simulink model "MotorModelSteadyStateCharacteristics"  (R2015b)
settings: Solver=VariableStepAuto  StartTime=0.0  StopTime=2000  RelTol=1e-4
values from neighbouring files (symbols this model uses):
  R_winding = Vdc_nom/I_stall    (= 0.16724738676)    [MotorModel_Mabuchi_RS_540.m]
  Vdc = 9.6    [MotorModel_Mabuchi_RS_540.m]    (also in Params.m)
libraries: simulink x7, LocalLib x1
settings Model: Creator=jje  LastModifiedBy=jje

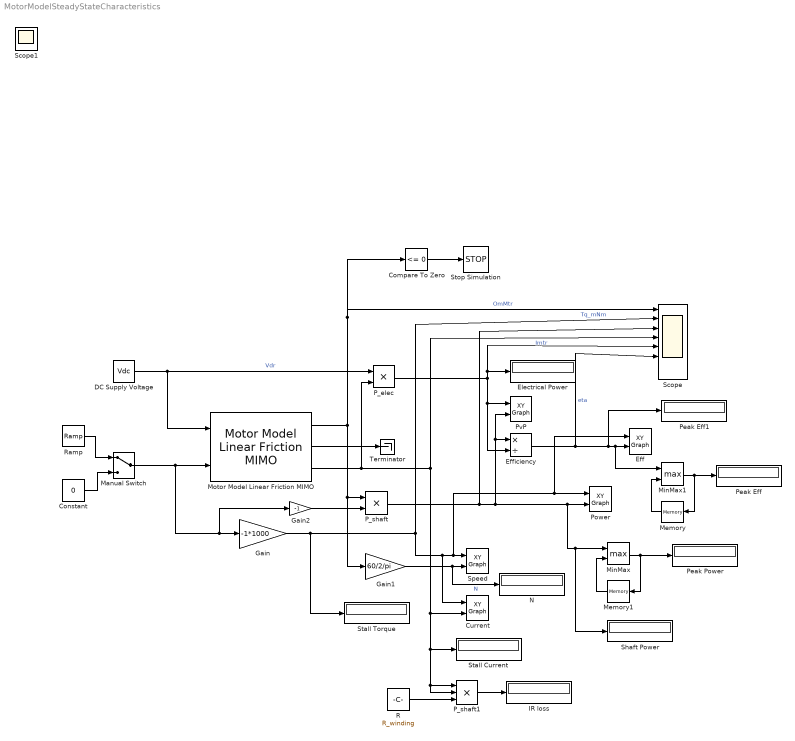
== system MotorModelSteadyStateCharacteristics ==
  Compare To Zero : simulink/Logic and Bit Operations/Compare To Zero  relop=<=  OutDataTypeStr=boolean
  Constant : Constant  Value=0
  Current : simulink/Sinks/XY Graph  xmin=0  xmax=225  ymin=0  ymax=60  st=0.01
  DC Supply Voltage : Constant  Value=Vdc
  Eff : simulink/Sinks/XY Graph  xmin=0  xmax=225  ymin=0  ymax=1  st=0.01
  Efficiency : Product  Inputs=*/
  Electrical Power : Display
  Gain : Gain  Gain=-1*1000
  Gain1 : Gain  Gain=60/2/pi
  Gain2 : Gain  Gain=-1
  IR loss : Display
  Manual Switch : ManualSwitch
  Memory : Memory
  Memory1 : Memory
  MinMax : MinMax  Function=max  Inputs=2
  MinMax1 : MinMax  Function=max  Inputs=2
  Motor Model Linear Friction MIMO : LocalLib/Motor Model Linear Friction MIMO
  N : Display
      settings: Format=decimal (Stored Integer)
  P_elec : Product
  P_shaft : Product
  P_shaft1 : Product  Inputs=3
  Peak Eff : Display
  Peak Eff1 : Display
  Peak Power : Display
  Power : simulink/Sinks/XY Graph  xmin=0  xmax=225  ymin=0  ymax=150  st=0.01
  PvP : simulink/Sinks/XY Graph  xmin=0  xmax=150  ymin=0  ymax=150  st=0.01
  R : Constant  Value=R_winding
  Ramp : simulink/Sources/Ramp  slope=-0.220/30  start=0.5  X0=0
  Scope : Scope  NumInputPorts=8
  Shaft Power : Display
  Speed : simulink/Sinks/XY Graph  xmin=0  xmax=225  ymin=0  ymax=30000  st=0.01
  Stall Current : Display
  Stall Torque : Display
  Stop Simulation : Stop
  Terminator : Terminator
  Scope1 : Scope
  wires:
  DC Supply Voltage/1 -> Motor Model Linear Friction MIMO/1, P_elec/1  "Vdr"
  Motor Model Linear Friction MIMO/1 -> Compare To Zero/1, Scope/1, P_shaft/1, Gain1/1  "OmMtr"
  Motor Model Linear Friction MIMO/3 -> P_elec/2, Scope/4, P_shaft1/2, P_shaft1/1, Stall Current/1, Current/2  "Imtr"
  Motor Model Linear Friction MIMO/2 -> Terminator/1
  Manual Switch/1 -> Motor Model Linear Friction MIMO/2, Gain2/1, Gain/1
  Compare To Zero/1 -> Stop Simulation/1
  Gain/1 -> Stall Torque/1, Scope/2, Current/1, Eff/1, Power/1, Speed/1  "Tq_mNm"
  Gain1/1 -> N/1, Speed/2  "N"
  P_shaft/1 -> PvP/2, Efficiency/1, Shaft Power/1, MinMax/1, Power/2, Scope/3
  P_elec/1 -> Efficiency/2, PvP/1, Electrical Power/1, Scope/5
  Efficiency/1 -> Scope/6, Peak Eff1/1, MinMax1/1, Eff/2  "eta"
  Gain2/1 -> P_shaft/2
  MinMax/1 -> Memory1/1, Peak Power/1
  Memory1/1 -> MinMax/2
  MinMax1/1 -> Memory/1, Peak Eff/1
  Memory/1 -> MinMax1/2
  Constant/1 -> Manual Switch/2
  Ramp/1 -> Manual Switch/1
  P_shaft1/1 -> IR loss/1
  R/1 -> P_shaft1/3
